simulink model "controller1_SR"  (R2020a)
settings: Solver=VariableStepAuto  StartTime=0.0  StopTime=30.0  RelTol=1e-3
values from neighbouring files (symbols this model uses):
  A = [0 1; -k/J -b/J]    [sofia_udp_test.m]
  B = [0; 1/J]    [sofia_udp_test.m]
  b = 0.05    [sofia_udp_test.m]
  C = [1 0]    [sofia_udp_test.m]
  D = zeros()    [sofia_udp_test.m]
  J = 0.0103    [capt_est_params.m]    (also in for_mat.m; sofia_udp_test.m = 0.0123)
  k = 0.1    [sofia_udp_test.m]
  omega_c = 62    [sofia_udp_test.m]
  Ts = mean(valid_dt)    [capt_est_params.m]    (also in capt_fidel_castro.m = mean(diff(time_data)); capt_id.m = mean(diff(time_data)); for_mat.m = mean(diff(seg_time)); sofia_udp_test.m = 0.001)
undefined symbols (not defined in the file or in its folder): den_d, Discrete, num_d, Time
libraries: simulink x1, ctrlSharedLib x1, SignalEditorBlockLib x1, etargetslib x1, instrumentlib x1
settings Model: Creator=javot  LastModifiedBy=javot

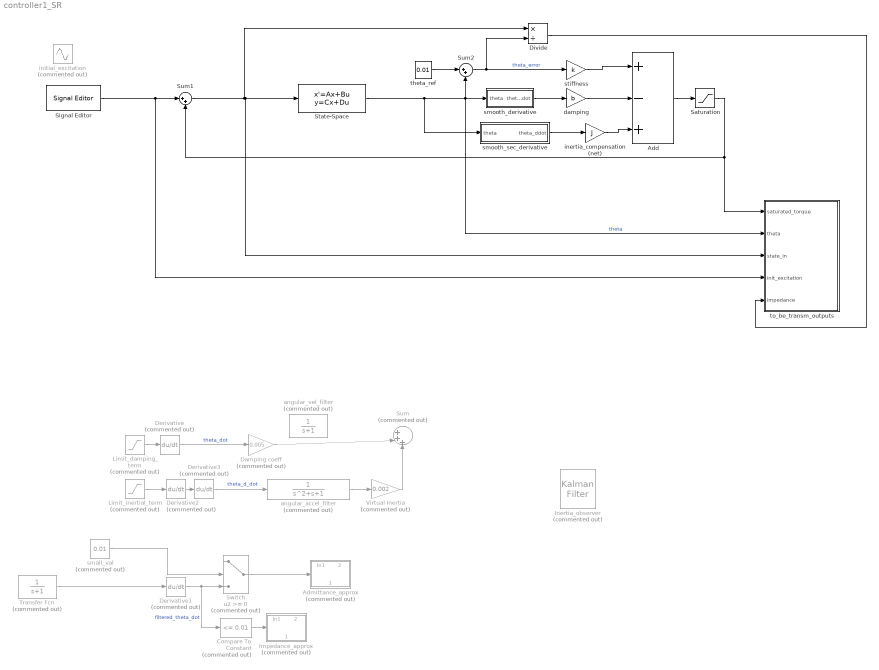
== system controller1_SR ==
  Add : Sum  Inputs=+-+
  Admittance_approx : Subsystem  Commented=on
  Compare To Constant : simulink/Logic and Bit Operations/Compare To Constant  Commented=on  relop=<=  const=0.01  OutDataTypeStr=boolean
  Damping coeff : Gain  Commented=on  Gain=0.005
  Derivative{,1..3} (4 alike) : Derivative  Commented=on
  Divide : Product  Inputs=*/
  Impedance_approx : Subsystem  Commented=on
  Inertia_observer : ctrlSharedLib/Kalman Filter  Commented=on  TimeDomain=Discrete-Time  UseCurrentEstimator=on  ModelSource=LTI State-Space Variable  ModelSourceVariable=ss(0.95,1,1,0,1)  A=0.95  B=1  C=1  D=0  NumberOfStates=1  NumberOfInputs=1  NumberOfOutputs=1  InitialEstimateSource=Dialog  X0=0  P0=10  UseK=off  UseGH=off  NumberOfProcessNoiseInputs=1  G=1  TimeInvariantG=on  H=0  TimeInvariantH=on  Q=0.05  TimeInvariantQ=on  R=1  TimeInvariantR=on  N=0  TimeInvariantN=on  AddInputPort=on  AddEnablePort=off  OutputEstimatedY=off  OutputP=off  Ts=-1
  Limit_damping_term : Saturate  Commented=on
  Limit_inertial_term : Saturate  Commented=on
  Saturation : Saturate  UpperLimit=1  LowerLimit=-1
  Signal Editor : SignalEditorBlockLib/Signal Editor  FileName=C:\Users\javot\Desktop\sofia_code\test_signals.mat  ActiveScenario=Scenario  ActiveSignal=Signal 1  IsBus=off  OutputBusObjectStr=Bus: BusObject  SampleTime=0.001  Interpolate=off  ZeroCross=off  OutputAfterFinalValue=Setting to zero  Unit=inherit  PreserveSignalName=on
  State-Space : StateSpace  A=A  B=B  C=C  D=D  InitialCondition=0  ContinuousStateAttributes="\"\""
  Sum : Sum  Commented=on  Inputs=|+++
  Sum1 : Sum  Inputs=|++
  Sum2 : Sum  Inputs=|++
  Switch : Switch  Commented=on  mask(TL_Switch){data={'date',740170.64219473384}}
      settings: CopyFcn=if exist('copy_tlblock') == 2, copy_tlblock(gcbh); end;  DeleteFcn=if exist('delete_tlblock','file')==2,delete_tlblock(gcbh);end  NameChangeFcn=if exist('rename_tlblock','file')==2,rename_tlblock(gcbh);end  OpenFcn=if exist('tl_open_blockdlg','file')==2,tl_open_blockdlg(gcbh);else,open_system(gcbh,'force');end
      mask Help: eval(['if exist(''tl_online_help'',''file'') == 2, tl_online_help(''Topic'',''TL_Switch''),else, web([''jar:file:///'',matlabroot,''/help/toolbox/simulink/help.jar!/slref/' lower(get_param(gcbh,'Blocktype')) '.html''], ''-helpbrowser''),end'])
      mask Display:
      | [x,y] = tlDrawBrandOnBlockIcon(gcbh);
      | plot(x,y);
  Transfer Fcn : TransferFcn  Commented=on  Denominator=[1 1]
  Virtual Inertia : Gain  Commented=on  Gain=0.002
  angular_accel_filter : TransferFcn  Commented=on  Denominator=[1 1 1]
  angular_vel_filter : TransferFcn  Commented=on  Denominator=[1 1]
  damping : Gain  Gain=b
  inertia_compensation (net) : Gain  Gain=J
  initial_excitation : Sin  Commented=on  SampleTime=Ts
  small_val : Constant  Commented=on  Value=0.01
  smooth_derivative : Subsystem
  smooth_sec_derivative : Subsystem
  stiffness : Gain  Gain=k
  theta_ref : Constant  Value=0.01
  to_be_transm_outputs : Subsystem
  wires:
  small_val/1 -> Switch/2
  Compare To Constant/1 -> Impedance_approx/Enable
  Switch/1 -> Admittance_approx/Enable
  Transfer Fcn/1 -> Derivative1/1
  Derivative2/1 -> Derivative3/1
  Virtual Inertia/1 -> Sum/3
  Damping coeff/1 -> Sum/2
  Limit_damping_term/1 -> Derivative/1
  Derivative1/1 -> Compare To Constant/1, Switch/3  "filtered_theta_dot"
  Limit_inertial_term/1 -> Derivative2/1
  angular_accel_filter/1 -> Virtual Inertia/1
  Derivative/1 -> Damping coeff/1  "theta_dot"
  Derivative3/1 -> angular_accel_filter/1  "theta_d_dot"
  State-Space/1 -> to_be_transm_outputs/2(theta), smooth_derivative/1(theta), Sum2/2, smooth_sec_derivative/1(theta)  "theta"
  theta_ref/1 -> Sum2/1
  Sum2/1 -> Divide/2, stiffness/1  "theta_error"
  stiffness/1 -> Add/1
  damping/1 -> Add/2
  inertia_compensation (net)/1 -> Add/3
  smooth_derivative/1(theta_dot) -> damping/1
  smooth_sec_derivative/1(theta_ddot) -> inertia_compensation (net)/1
  Sum1/1 -> to_be_transm_outputs/3(state_in), State-Space/1, Divide/1
  Divide/1 -> to_be_transm_outputs/5(impedance)
  Add/1 -> Saturation/1
  Saturation/1 -> Sum1/2, to_be_transm_outputs/1(saturated_torque)
  Signal Editor/1 -> to_be_transm_outputs/4(init_excitation), Sum1/1

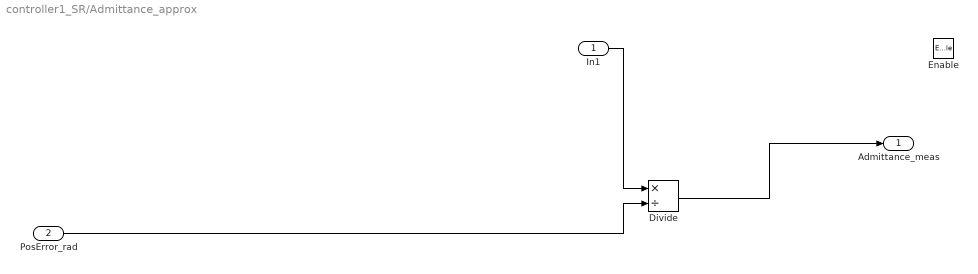
== system controller1_SR/Admittance_approx ==
  In1 : Inport
  PosError_rad : Inport  Port=2
  Enable : EnablePort
  Divide : Product  Inputs=*/
  Admittance_meas : Outport
  wires:
  Divide/1 -> Admittance_meas/1
  PosError_rad/1 -> Divide/2
  In1/1 -> Divide/1

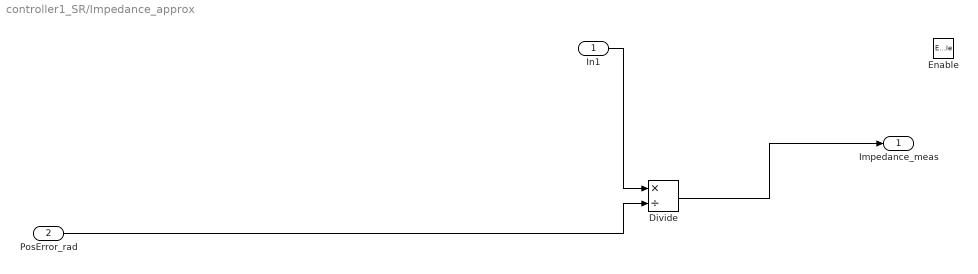
== system controller1_SR/Impedance_approx ==
  In1 : Inport
  PosError_rad : Inport  Port=2
  Enable : EnablePort
  Divide : Product  Inputs=*/
  Impedance_meas : Outport
  wires:
  Divide/1 -> Impedance_meas/1
  PosError_rad/1 -> Divide/2
  In1/1 -> Divide/1

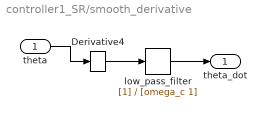
== system controller1_SR/smooth_derivative ==
  theta : Inport
  Derivative4 : Derivative
  low_pass_filter : TransferFcn  Denominator=[omega_c 1]
  theta_dot : Outport
  wires:
  Derivative4/1 -> low_pass_filter/1
  theta/1 -> Derivative4/1
  low_pass_filter/1 -> theta_dot/1

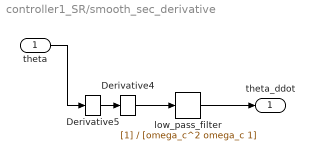
== system controller1_SR/smooth_sec_derivative ==
  theta : Inport
  Derivative4 : Derivative
  Derivative5 : Derivative
  low_pass_filter : TransferFcn  Denominator=[omega_c^2 omega_c 1]
  theta_ddot : Outport
  wires:
  Derivative5/1 -> Derivative4/1
  Derivative4/1 -> low_pass_filter/1
  theta/1 -> Derivative5/1
  low_pass_filter/1 -> theta_ddot/1

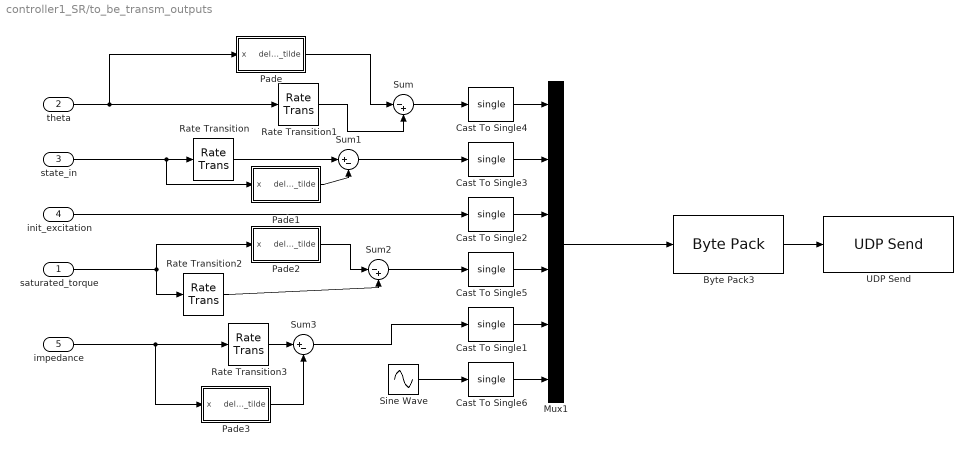
== system controller1_SR/to_be_transm_outputs ==
  saturated_torque : Inport
  theta : Inport  Port=2
  state_in : Inport  Port=3
  init_excitation : Inport  Port=4
  impedance : Inport  Port=5
  Byte Pack3 : etargetslib/Byte Pack  datatypes={'single'}  byteAlign=1
  Cast To Single{1..6} (6 alike) : DataTypeConversion  OutDataTypeStr=single
  Mux1 : Mux  Inputs=6
  Pade : Subsystem
  Pade1 : Subsystem
  Pade2 : Subsystem
  Pade3 : Subsystem
  Rate Transition{,1..3} (4 alike) : RateTransition
  Sine Wave : Sin  SampleTime=0.001
  Sum : Sum  Inputs=|-+
  Sum1 : Sum  Inputs=|+-
  Sum2 : Sum  Inputs=|-+
  Sum3 : Sum  Inputs=|+-
  UDP Send : instrumentlib/UDP Send  Host=134.105.60.99  Port=55001  LocalPort=-1  EnablePortSharing=off  ByteOrder=BigEndian  OutputDatagramPacketSize=512  EnableBlockingMode=on  LocalAddress=0.0.0.0
  wires:
  Byte Pack3/1 -> UDP Send/1
  Mux1/1 -> Byte Pack3/1
  Sine Wave/1 -> Cast To Single6/1
  init_excitation/1 -> Cast To Single2/1
  theta/1 -> Pade/1(x), Rate Transition1/1
  saturated_torque/1 -> Pade2/1(x), Rate Transition2/1
  impedance/1 -> Pade3/1(x), Rate Transition3/1
  Cast To Single4/1 -> Mux1/1
  Cast To Single3/1 -> Mux1/2
  Cast To Single5/1 -> Mux1/4
  Cast To Single2/1 -> Mux1/3
  Cast To Single1/1 -> Mux1/5
  Cast To Single6/1 -> Mux1/6
  Rate Transition1/1 -> Sum/2
  Sum/1 -> Cast To Single4/1
  Rate Transition/1 -> Sum1/1
  Sum1/1 -> Cast To Single3/1
  Rate Transition2/1 -> Sum2/2
  Sum2/1 -> Cast To Single5/1
  Rate Transition3/1 -> Sum3/1
  Sum3/1 -> Cast To Single1/1
  state_in/1 -> Pade1/1(x), Rate Transition/1
  Pade2/1(delay_tilde) -> Sum2/1
  Pade/1(delay_tilde) -> Sum/1
  Pade1/1(delay_tilde) -> Sum1/2
  Pade3/1(delay_tilde) -> Sum3/2

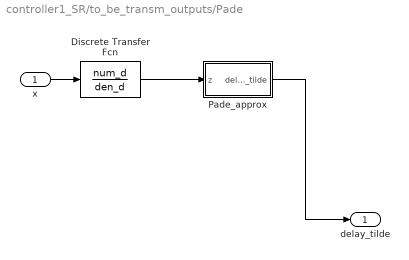
== system controller1_SR/to_be_transm_outputs/Pade ==
  x : Inport
  Discrete Transfer Fcn : DiscreteTransferFcn  Numerator=num_d  Denominator=den_d
  Pade_approx : MATLAB Function  TreatAsAtomicUnit=on
  delay_tilde : Outport
  wires:
  Discrete Transfer Fcn/1 -> Pade_approx/1(z)
  Pade_approx/1(delay_tilde) -> delay_tilde/1
  x/1 -> Discrete Transfer Fcn/1

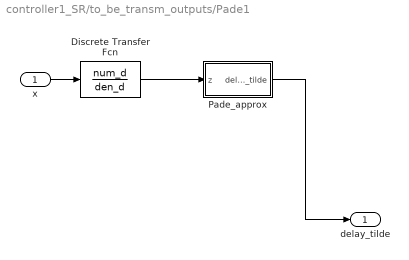
== system controller1_SR/to_be_transm_outputs/Pade1 ==
  x : Inport
  Discrete Transfer Fcn : DiscreteTransferFcn  Numerator=num_d  Denominator=den_d
  Pade_approx : MATLAB Function  TreatAsAtomicUnit=on
  delay_tilde : Outport
  wires:
  Discrete Transfer Fcn/1 -> Pade_approx/1(z)
  Pade_approx/1(delay_tilde) -> delay_tilde/1
  x/1 -> Discrete Transfer Fcn/1

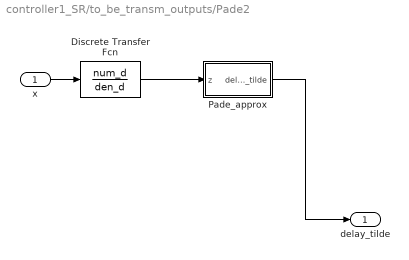
== system controller1_SR/to_be_transm_outputs/Pade2 ==
  x : Inport
  Discrete Transfer Fcn : DiscreteTransferFcn  Numerator=num_d  Denominator=den_d
  Pade_approx : MATLAB Function  TreatAsAtomicUnit=on
  delay_tilde : Outport
  wires:
  Discrete Transfer Fcn/1 -> Pade_approx/1(z)
  Pade_approx/1(delay_tilde) -> delay_tilde/1
  x/1 -> Discrete Transfer Fcn/1

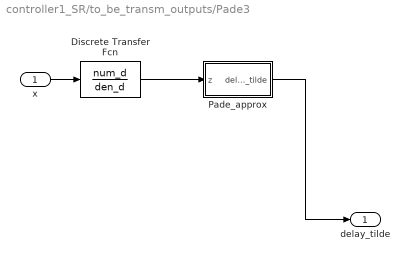
== system controller1_SR/to_be_transm_outputs/Pade3 ==
  x : Inport
  Discrete Transfer Fcn : DiscreteTransferFcn  Numerator=num_d  Denominator=den_d
  Pade_approx : MATLAB Function  TreatAsAtomicUnit=on
  delay_tilde : Outport
  wires:
  Discrete Transfer Fcn/1 -> Pade_approx/1(z)
  Pade_approx/1(delay_tilde) -> delay_tilde/1
  x/1 -> Discrete Transfer Fcn/1

== matlab function controller1_SR/to_be_transm_outputs/Pade/Pade_approx ==
  data: delay_tilde output; z input
function delay_tilde= fcn(z)
persistent z_prev; 
persistent delay_prev;

if isempty(z_prev)
    z_prev = 0;
    delay_prev = 0;
end
delay_tilde = z/3 + z_prev + (1/3)*delay_prev;
z_prev = z;
delay_prev = delay_tilde;

end

== matlab function controller1_SR/to_be_transm_outputs/Pade2/Pade_approx ==
  data: delay_tilde output; z input
function delay_tilde= fcn(z)
persistent z_prev; 
persistent delay_prev;

if isempty(z_prev)
    z_prev = 0;
    delay_prev = 0;
end
delay_tilde = z/3 + z_prev + (1/3)*delay_prev;
z_prev = z;
delay_prev = delay_tilde;

end

== matlab function controller1_SR/to_be_transm_outputs/Pade3/Pade_approx ==
  data: delay_tilde output; z input
function delay_tilde= fcn(z)
persistent z_prev; 
persistent delay_prev;

if isempty(z_prev)
    z_prev = 0;
    delay_prev = 0;
end
delay_tilde = z/3 + z_prev + (1/3)*delay_prev;
z_prev = z;
delay_prev = delay_tilde;

end

== matlab function controller1_SR/to_be_transm_outputs/Pade1/Pade_approx ==
  data: delay_tilde output; z input
function delay_tilde= fcn(z)
persistent z_prev; 
persistent delay_prev;

if isempty(z_prev)
    z_prev = 0;
    delay_prev = 0;
end
delay_tilde = z/3 + z_prev + (1/3)*delay_prev;
z_prev = z;
delay_prev = delay_tilde;

end
